simulink model "btp_VERSION2_draft1"  (R2020a)
settings: Solver=VariableStepAuto  StartTime=0.0  StopTime=1e5  RelTol=1e-3
PreLoadFcn:
  | building_length = 15; % m
  | building_width = 10; % m
  | building_height = 2.5; % m
  | 
  | wall_thickness = 0.2; % m
  | wall_density = 2000; % kg/m^3
  | wall_specific_heat = 840; % J/(kg*K)
  | wall_conductivity = 0.04; % W/(m*K)
  | wall_heat_transfer_coeff_internal = 25; % W/(m^2*K)
  | wall_heat_transfer_coeff_external = 35; % W/(m^2*K)
  | 
  | roof_thickness = 0.2; % m
  | roof_density = 2000; % kg/m^3
  | roof_specific_heat = 840; % J/(kg*K)
  | roof_conductivity = 0.035; % W/(m*K)
  | roof_heat_transfer_coeff_internal = 10; % W/(m^2*K)
  | roof_heat_transfer_coeff_external = 30; % W/(m^2*K)
  | 
  | floor_thickness = 0.1; % m
  | floor_conductivity = 0.15; % W/(m*K)
  | floor_heat_transfer_coeff_internal = 15; % W/(m^2*K)
  | 
  | door_area = 2*0.6; % m^2
  | 
  | duct_area = 0.1^2; % m^2
  | 
  | fan_setting_table = 0 : 4; % 1
  | fan_flow_rate_table = [0 0.08 0.12 0.16 0.2]; % kg/s
  | 
  | initial_temperature = 35; % degC
  | ground_temperature = 25; % degC
  | 
  | flow_reversal_Mach = 1e-5; % 1
InitFcn:
  | zone_volume = building_length * building_width * building_height / 4; % m^3
  | zone_flow_area = 0.7 * building_height * (building_length + building_width) / 4; % m^2
model workspace (MAT data in the model file):
  CO2_occupant = 0.01
  N_occupant = 1
  T_occupant = 30
  W_occupant = 70
  y_co2_env = 0.04
undefined symbols (not defined in the file): mdot_coolant, sigbuilder_block, T_coolant
libraries: fl_lib x57, nesl_utility x23, HVAC_lib x1
(part 1 of 2)
CloseFcn:
  | try,close(h1_ssc_building_ventilation),end
  | clear h1_ssc_building_ventilation
  | try,close(h2_ssc_building_ventilation),end
  | clear h2_ssc_building_ventilation
  | try,close(h3_ssc_building_ventilation),end
  | clear h3_ssc_building_ventilation
  | try,close(h4_ssc_building_ventilation),end
  | clear h4_ssc_building_ventilation
  | 
  | clear simlog_ssc_building_ventilation tout
  | 
  | clear building_length building_width building_height zone_volume zone_flow_area
  | clear wall_thickness wall_density wall_specific_heat wall_conductivity wall_heat_transfer_coeff_internal wall_heat_transfer_coeff_external
  | clear roof_thickness roof_density roof_specific_heat roof_conductivity roof_heat_transfer_coeff_internal roof_heat_transfer_coeff_external
  | clear floor_thickness floor_conductivity floor_heat_transfer_coeff_internal
  | clear door_area duct_area fan_setting_table fan_flow_rate_table initial_temperature ground_temperature flow_reversal_Mach
Description:
  | Building Ventilation
settings Model: Creator=MathWorks  LastModifiedBy=PRANAV REDDY
settings DataIOCC: ReturnWorkspaceOutputs=off
settings DebuggingCC: PregeneratedLibrarySubsystemCodeDiagnostic=none  ArithmeticOperatorsInVariantConditions=warning
settings SFSimCC: SimUseLocalCustomCode=off  CustomCodeUndefinedFunction=UseInterfaceOnly
settings RTWCC: RTWUseLocalCustomCode=off
settings CodeAppCC: StateflowObjectComments=on
settings SimscapeCC: SimscapeLogType=all  SimscapeLogSimulationStatistics=on  SimscapeLogName=simlog_ssc_building_ventilation  SimscapeLogDataHistory=10000

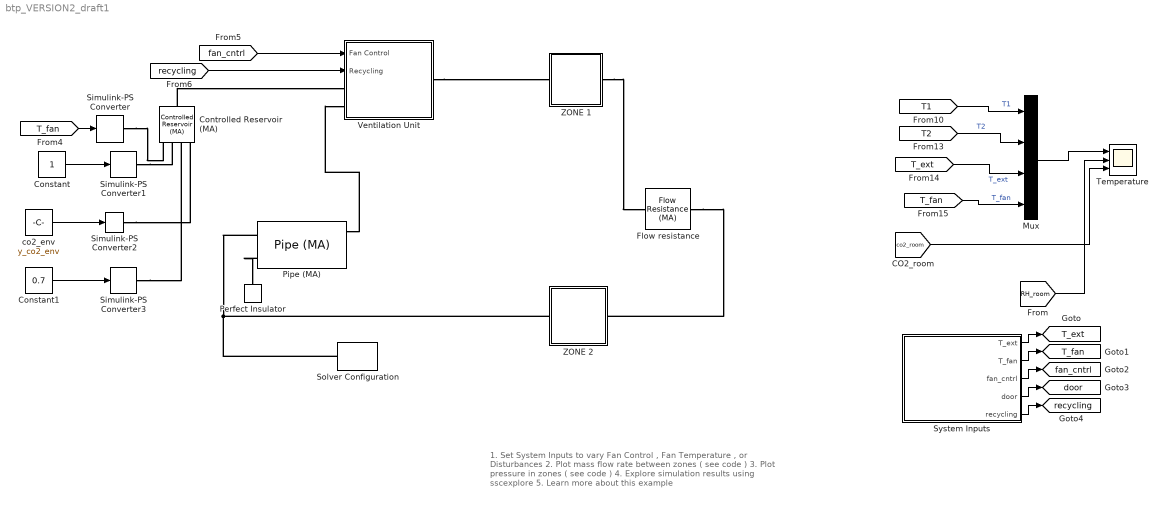
== system btp_VERSION2_draft1 ==
  note: 1. Set System Inputs to vary Fan Control , Fan Temperature , or Disturbances
      | 2. Plot mass flow rate between zones ( see code )
      | 3. Plot pressure in zones ( see code )
      | 4. Explore simulation results using sscexplore
      | 5. Learn more about this example
  Constant : Constant
  Constant1 : Constant  Value=0.7
  Controlled Reservoir (MA) : fl_lib/Moist Air/Elements/Controlled Reservoir (MA)  moisture_spec=foundation.enum.moisture_spec.relative_humidity  trace_gas_spec=foundation.enum.trace_gas_spec.mole_fraction  RH_ws=1  area_A=duct_area m^2  input_error_spec=foundation.enum.input_range_error.warn
      settings: SourceProductBaseCode=SS  InternalSimscapePortConfiguration="{\"Bottom\":[],\"Left\":[{\"id\":\"A\",\"label\":\"A\",\"type\":\"foundation.moist_air.moist_air\"}],\"Right\":[{\"id\":\"T\",\"label\":\"T\",\"type\":\"input\"},{\"id\":\"P\",\"label\":\"P\",\"type\":\"input\"},{\"id\":\"W\",\"label\":\"W\",\"type\":\"input\"},{\"id\":\"G\",\"label\":\"G\",\"type\":\"input\"}],\"Top\":[]}"
  Flow resistance : fl_lib/Moist Air/Elements/Flow Resistance (MA)  delta_p_nominal=20 Pa  mdot_nominal=0.04 kg/s  rho_nominal=1.2 kg/m^3  area=zone_flow_area m^2  laminar_fraction=1e-3
      settings: SourceProductBaseCode=SS
  Mux : Mux
  Perfect Insulator : fl_lib/Thermal/Thermal Elements/Perfect Insulator  T_specify=off  T_priority=None  T=0 K  T_nominal_specify=off  T_nominal_unit=K  T_nominal_value=1
  Pipe (MA) : fl_lib/Moist Air/Elements/Pipe (MA)  length=building_length + building_width m  area=duct_area m^2  Dh=sqrt(duct_area) m  length_add=0 m  roughness=15e-6 m  Re_lam=2000  Re_tur=4000  shape_factor=56.92  Nu_lam=2.98  RH_ws=1  time_constant=1e-3 s  moisture_trace_gas_source=foundation.enum.moisture_trace_gas_source.none  moisture_source_spec=foundation.enum.moisture_source_spec.vapor  moisture_mass_flow=0 kg/s  moisture_temperature_spec=foundation.enum.temperature_spec.atmospheric  moisture_temperature=293.15 K  trace_gas_mass_flow=0 kg/s  trace_gas_temperature_spec=foundation.enum.temperature_spec.atmospheric  trace_gas_temperature=293.15 K  p_I_specify=off  p_I_priority=High  p_I=0.101325 MPa  p_I_nominal_specify=off  p_I_nominal_unit=MPa  p_I_nominal_value=1  T_I_specify=off  T_I_priority=High  T_I=293.15 K  T_I_nominal_specify=off  T_I_nominal_unit=K  T_I_nominal_value=1  RH_I_specify=off  RH_I_priority=High  RH_I=0  RH_I_nominal_specify=off  RH_I_nominal_unit=1  RH_I_nominal_value=1  x_w_I_specify=off  x_w_I_priority=None  x_w_I=0  x_w_I_nominal_specify=off  x_w_I_nominal_unit=1  x_w_I_nominal_value=1  y_w_I_specify=off  y_w_I_priority=None  y_w_I=0  y_w_I_nominal_specify=off  y_w_I_nominal_unit=1  y_w_I_nominal_value=1  HR_I_specify=off  HR_I_priority=None  HR_I=0  HR_I_nominal_specify=off  HR_I_nominal_unit=1  HR_I_nominal_value=1  x_g_I_specify=off  x_g_I_priority=High  x_g_I=0  x_g_I_nominal_specify=off  x_g_I_nominal_unit=1  x_g_I_nominal_value=1  y_g_I_specify=off  y_g_I_priority=None  y_g_I=0  y_g_I_nominal_specify=off  y_g_I_nominal_unit=1  y_g_I_nominal_value=1
      settings: SourceProductBaseCode=SS
  Simulink-PS Converter : nesl_utility/Simulink-PS Converter  PhysicalDomain=network_engine_domain  SubClassName=ps_input  LeftPortType=input  RightPortType=output  PseudoPeriodic=off  Frequencies=[]  NoiseDistribution=none  NoiseParameters=[]  Unit=degC  AffineConversion=on  FilteringAndDerivatives=provide  SimscapeFilterOrder=1  InputFilterTimeConstant=0.001  UdotUserProvided=0
  Simulink-PS Converter1 : nesl_utility/Simulink-PS Converter  PhysicalDomain=network_engine_domain  SubClassName=ps_input  LeftPortType=input  RightPortType=output  PseudoPeriodic=off  Frequencies=[]  NoiseDistribution=none  NoiseParameters=[]  Unit=atm  AffineConversion=off  FilteringAndDerivatives=provide  SimscapeFilterOrder=1  InputFilterTimeConstant=0.001  UdotUserProvided=0
  Simulink-PS Converter2 : nesl_utility/Simulink-PS Converter  PhysicalDomain=network_engine_domain  SubClassName=ps_input  LeftPortType=input  RightPortType=output  PseudoPeriodic=off  Frequencies=[]  NoiseDistribution=none  NoiseParameters=[]  Unit=1  AffineConversion=off  FilteringAndDerivatives=provide  SimscapeFilterOrder=1  InputFilterTimeConstant=0.001  UdotUserProvided=0
  Simulink-PS Converter3 : nesl_utility/Simulink-PS Converter  PhysicalDomain=network_engine_domain  SubClassName=ps_input  LeftPortType=input  RightPortType=output  PseudoPeriodic=off  Frequencies=[]  NoiseDistribution=none  NoiseParameters=[]  Unit=1  AffineConversion=off  FilteringAndDerivatives=provide  SimscapeFilterOrder=1  InputFilterTimeConstant=0.001  UdotUserProvided=0
  Solver Configuration : nesl_utility/Solver Configuration  PhysicalDomain=network_engine_domain  SubClassName=solver  LeftPortType=input  RightPortType=generic  Tones=[]  Harmonics=[]  SimulateNoise=off  Profile=off  UseLocalSampling=off  EnableSwitchedLinearOptims=on  FrequencyDomain=off  UseCCode=off  RelTol=0.001  AbsTol=1e-06  MinStep=1e-09  ToWorkspace=off  RevertToSquareIcSolve=off  NumHomotopyIterations=100  PhasorMode=off  PhasorModeNumHarmonics=1  DoDC=off  ResidualTolerance=1e-9  UseLocalSolver=off  LocalSolverChoice=NE_BACKWARD_EULER_ADVANCER  LocalSolverSampleTime=0.05  DoFixedCost=off  MaxNonlinIter=3  MaxModeIter=2  LinearAlgebra=auto  EquationFormulation=NE_TIME_EF  DelaysMemoryBudget=1024  AutomaticFiltering=on  FilteringTimeConstant=0.001  PartitionStorageMethod=AS_NEEDED  PartitionMemoryBudget=1024  PartitionMethod=FAST
  System Inputs : Subsystem  Tag=STV Subsys  LoadFcn=sigbuilder_block('load');  StartFcn=sigbuilder_block('start');  StopFcn=sigbuilder_block('stop');  ClipboardFcn=sigbuilder_block('clipboard');  mask(Sigbuilder block){tuvar=[0:10]}
      mask help: Simulink:masks:SigbuilderBlock_MD
      mask init:
      | if ~strcmp(get_param(bdroot(gcbh),'SimulationStatus'),'stopped') tuvar = sigbuilder_block('maskInit'); end
      settings: CopyFcn=sigbuilder_block('copy');  DeleteFcn=sigbuilder_block('delete');  ModelCloseFcn=sigbuilder_block('modelClose');  PreSaveFcn=sigbuilder_block('preSave');  PauseFcn=sigbuilder_block('pause');  ContinueFcn=sigbuilder_block('continue');  NameChangeFcn=sigbuilder_block('namechange');  OpenFcn=sigbuilder_block('open',[96 153 550.5 359.25 ]);  CloseFcn=sigbuilder_block('close');
      mask Display: plot(0, 0, 100, 100,[2, 2, 32, 32, 2], [68, 8, 8, 68, 68],[32, 2], [38, 38], [32, 19, 2],[53, 60, 44], [32, 17, 17, 2],[16, 16, 31, 31]);txt = getActiveGroup(gcbh);text(2, 100, txt,'verticalAlignment', 'top');
  Temperature : Scope  NumInputPorts=3
  Ventilation Unit : Subsystem  Tag=PublishSubsystem
  ZONE 1 : Subsystem
  ZONE 2 : Subsystem
  co2_env : Constant  Value=y_co2_env
  tag scope: T_ext=global, T_fan=global, door=global, fan_cntrl=global, recycling=global
  wires:
  Constant/1 -> Simulink-PS Converter1/1
  [T_fan] -> Simulink-PS Converter/1
  [fan_cntrl] -> Ventilation Unit/1(Fan Control)
  [recycling] -> Ventilation Unit/2(Recycling)
  System Inputs/1(T_ext) -> [T_ext]
  System Inputs/2(T_fan) -> [T_fan]
  System Inputs/3(fan_cntrl) -> [fan_cntrl]
  System Inputs/4(door) -> [door]
  System Inputs/5(recycling) -> [recycling]
  [T1] -> Mux/1  "T1"
  [T2] -> Mux/2  "T2"
  [T_ext] -> Mux/3  "T_ext"
  [T_fan] -> Mux/4  "T_fan"
  Mux/1 -> Temperature/1
  co2_env/1 -> Simulink-PS Converter2/1
  [co2_room] -> Temperature/3
  Constant1/1 -> Simulink-PS Converter3/1
  [RH_room] -> Temperature/2
  connections:
  Simulink-PS Converter/RConn1 -- Controlled Reservoir (MA)/RConn1
  Simulink-PS Converter1/RConn1 -- Controlled Reservoir (MA)/RConn2
  Controlled Reservoir (MA)/LConn1 -- Ventilation Unit/LConn1
  Pipe (MA)/RConn1 -- Ventilation Unit/LConn2
  Pipe (MA)/LConn2 -- Perfect Insulator/LConn1
  Solver Configuration/RConn1 -- Pipe (MA)/LConn1 -- ZONE 2/LConn1
  Flow resistance/RConn1 -- ZONE 2/RConn1
  ZONE 1/RConn1 -- Flow resistance/LConn1
  Ventilation Unit/RConn1 -- ZONE 1/LConn1
  Simulink-PS Converter2/RConn1 -- Controlled Reservoir (MA)/RConn4
  Simulink-PS Converter3/RConn1 -- Controlled Reservoir (MA)/RConn3

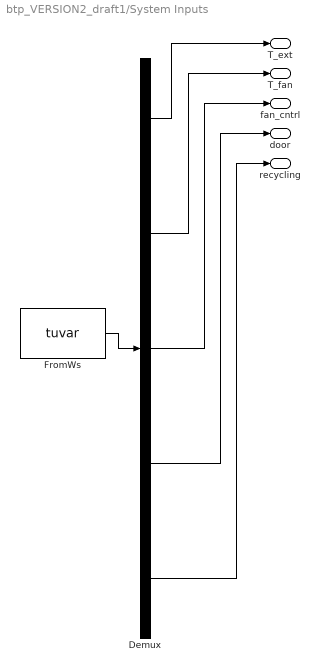
== system btp_VERSION2_draft1/System Inputs ==
  Demux : Demux  Tag=STV Demux  Outputs=5
      settings: DisplayOption=none
  FromWs : FromWorkspace  Tag=STV FromWs  VariableName=tuvar
      SigBuilderData=|
      | common.afterFinalStr = 'Extrapolate'
      | common.sampleTime = 0
      | dataSet(1).timeRange = [0 100000]
      | dataSet(1).name = 'Fan Control'
      | dataSet(2).timeRange = [0 100000]
      | dataSet(2).name = 'Fan Temperature'
      | dataSet(3).timeRange = [0 100000]
      | dataSet(3).name = 'Disturbances'
      | sbobj.Groups(1).Name = 'Fan Control'
      | sbobj.Groups(1).Signals(1).Name = 'T_ext'
      | sbobj.Groups(1).Signals(1).XData = [0 100000]
      | sbobj.Groups(1).Signals(1).YData = [35 35]
      | sbobj.Groups(1).Signals(2).Name = 'T_fan'
      | sbobj.Groups(1).Signals(2).XData = [0 100000]
      | sbobj.Groups(1).Signals(2).YData = [20 20]
      | sbobj.Groups(1).Signals(3).Name = 'fan_cntrl'
      | sbobj.Groups(1).Signals(3).XData = [0 20000 20000 40000 40000 60000 60000 80000 80000 100000]
      | sbobj.Groups(1).Signals(3).YData = [1 1 2 2 1 1 0 0 1 1]
      | sbobj.Groups(1).Signals(4).Name = 'door'
      | sbobj.Groups(1).Signals(4).XData = [0 100000]
      | sbobj.Groups(1).Signals(4).YData = [0 0]
      | sbobj.Groups(1).Signals(5).Name = 'recycling'
      | sbobj.Groups(1).Signals(5).XData = [0 100000]
      | sbobj.Groups(1).Signals(5).YData = [0 0]
      | sbobj.Groups(1).TimeRange = [0 100000]
      | sbobj.Groups(2).Name = 'Fan Temperature'
      | sbobj.Groups(2).Signals(1).Name = 'T_ext'
      | sbobj.Groups(2).Signals(1).XData = [0 100000]
      | sbobj.Groups(2).Signals(1).YData = [35 35]
      | sbobj.Groups(2).Signals(2).Name = 'T_fan'
      | sbobj.Groups(2).Signals(2).XData = [0 20000 40000 60000 80000 100000]
      | sbobj.Groups(2).Signals(2).YData = [20 20 20 20 20 20]
      | sbobj.Groups(2).Signals(3).Name = 'fan_cntrl'
      | sbobj.Groups(2).Signals(3).XData = [0 100000]
      | sbobj.Groups(2).Signals(3).YData = [1 1]
      | sbobj.Groups(2).Signals(4).Name = 'door'
      | sbobj.Groups(2).Signals(4).XData = [0 24200 34000 43600 100000]
      | sbobj.Groups(2).Signals(4).YData = [0 0 1.1 0 0]
      | sbobj.Groups(2).Signals(5).Name = 'recycling'
      | sbobj.Groups(2).Signals(5).XData = [0 20400 20400 78000 78000 100000]
      | sbobj.Groups(2).Signals(5).YData = [0 0 1 1 0 0]
      | sbobj.Groups(2).TimeRange = [0 100000]
      | sbobj.Groups(3).Name = 'Disturbances'
      | sbobj.Groups(3).Signals(1).Name = 'T_ext'
      | sbobj.Groups(3).Signals(1).XData = [0 100000]
      | sbobj.Groups(3).Signals(1).YData = [33.8 33.8]
      | sbobj.Groups(3).Signals(2).Name = 'T_fan'
      | sbobj.Groups(3).Signals(2).XData = [0 100000]
      | sbobj.Groups(3).Signals(2).YData = [21 21]
      | sbobj.Groups(3).Signals(3).Name = 'fan_cntrl'
      | sbobj.Groups(3).Signals(3).XData = [0 100000]
      | sbobj.Groups(3).Signals(3).YData = [1 1]
      | sbobj.Groups(3).Signals(4).Name = 'door'
      | sbobj.Groups(3).Signals(4).XData = [0 20000 30000 40000 100000]
      | sbobj.Groups(3).Signals(4).YData = [0 0 1 0 0]
      | sbobj.Groups(3).Signals(5).Name = 'recycling'
      | sbobj.Groups(3).Signals(5).XData = [0 65800 65800 95400 95400 100000]
      | sbobj.Groups(3).Signals(5).YData = [0 0 1 1 0 0]
      | sbobj.Groups(3).TimeRange = [0 100000]
  T_ext : Outport  Tag=STV Outport  VectorParamsAs1DForOutWhenUnconnected=off
  T_fan : Outport  Tag=STV Outport  Port=2  VectorParamsAs1DForOutWhenUnconnected=off
  fan_cntrl : Outport  Tag=STV Outport  Port=3  VectorParamsAs1DForOutWhenUnconnected=off
  door : Outport  Tag=STV Outport  Port=4  VectorParamsAs1DForOutWhenUnconnected=off
  recycling : Outport  Tag=STV Outport  Port=5  VectorParamsAs1DForOutWhenUnconnected=off
  wires:
  FromWs/1 -> Demux/1
  Demux/1 -> T_ext/1
  Demux/2 -> T_fan/1
  Demux/3 -> fan_cntrl/1
  Demux/4 -> door/1
  Demux/5 -> recycling/1

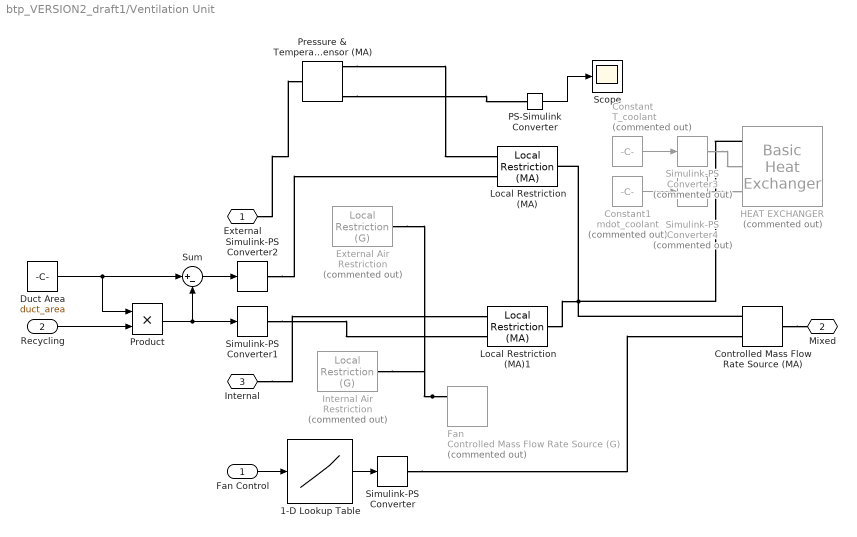
== system btp_VERSION2_draft1/Ventilation Unit ==
  Fan Control : Inport
  Recycling : Inport  Port=2
  1-D Lookup Table : Lookup_n-D  NumberOfTableDimensions=1  BreakpointsForDimension1=fan_setting_table  Table=fan_flow_rate_table  ExtrapMethod=Clip  InternalRulePriority=Speed  RndMeth=Simplest  InputSameDT=on
  Constant : Constant  Commented=on  Value=T_coolant
  Constant1 : Constant  Commented=on  Value=mdot_coolant
  Controlled Mass Flow Rate Source (MA) : fl_lib/Moist Air/Sources/Controlled Mass Flow Rate Source (MA)  power_spec=foundation.enum.power_spec.isentropic  area_A=duct_area m^2  area_B=duct_area m^2
      settings: SourceProductBaseCode=SS  InternalSimscapePortConfiguration="{\"Bottom\":[],\"Left\":[{\"id\":\"A\",\"label\":\"A\",\"type\":\"foundation.moist_air.moist_air\"},{\"id\":\"M\",\"label\":\"M\",\"type\":\"input\"}],\"Right\":[{\"id\":\"B\",\"label\":\"B\",\"type\":\"foundation.moist_air.moist_air\"}],\"Top\":[]}"
  Duct Area : Constant  Value=duct_area
  External Air Restriction : fl_lib/Gas/Elements/Local Restriction (G)  Commented=on  restriction_type=foundation.enum.restriction_type.variable  restriction_area=1e-3 m^2  min_area=1e-10 m^2  max_area=0.99 * duct_area m^2  area=duct_area m^2  Cd=0.8  B_lam=0.999
      settings: SourceProductBaseCode=SS  InternalSimscapePortConfiguration="{\"Bottom\":[],\"Left\":[{\"id\":\"A\",\"label\":\"A\",\"type\":\"foundation.gas.gas\"},{\"id\":\"area_in\",\"label\":\"AR\",\"type\":\"input\"}],\"Right\":[{\"id\":\"B\",\"label\":\"B\",\"type\":\"foundation.gas.gas\"}],\"Top\":[]}"
  Fan : fl_lib/Gas/Sources/Controlled Mass Flow Rate Source (G)  Commented=on  power_spec=1  area_A=duct_area m^2  area_B=duct_area m^2
      settings: SourceProductName=Foundation Library  InternalSimscapePortConfiguration="{\"Bottom\":[],\"Left\":[{\"id\":\"A\",\"label\":\"A\",\"type\":\"foundation.gas.gas\"},{\"id\":\"M\",\"label\":\"M\",\"type\":\"input\"}],\"Right\":[{\"id\":\"B\",\"label\":\"B\",\"type\":\"foundation.gas.gas\"}],\"Top\":[]}"
  HEAT EXCHANGER : HVAC_lib/Basic Heat Exchanger  Commented=on  Q_des=4.8 kW  T1_des=30 degC  mdot1_des=3 kg/s  cp1_des=1.8 kJ/kg/K  Dp1_des=0.2 kPa  T2_des=T_coolant degC  mdot2_des=mdot_coolant kg/s  cp2_des=10 kJ/kg/K  volume=1e-1 m^3  port_area=duct_area m^2  RH_ws=1  time_constant=1e-3 s  p_I_specify=on  p_I_priority=High  p_I=p_env MPa  p_I_nominal_specify=off  p_I_nominal_unit=MPa  p_I_nominal_value=1  T_I_specify=on  T_I_priority=High  T_I=T_init degC  T_I_nominal_specify=off  T_I_nominal_unit=K  T_I_nominal_value=1  RH_I_specify=on  RH_I_priority=High  RH_I=RH_init  RH_I_nominal_specify=off  RH_I_nominal_unit=1  RH_I_nominal_value=1  x_w_I_specify=off  x_w_I_priority=None  x_w_I=0  x_w_I_nominal_specify=off  x_w_I_nominal_unit=1  x_w_I_nominal_value=1  y_w_I_specify=off  y_w_I_priority=None  y_w_I=0  y_w_I_nominal_specify=off  y_w_I_nominal_unit=1  y_w_I_nominal_value=1  HR_I_specify=off  HR_I_priority=None  HR_I=0  HR_I_nominal_specify=off  HR_I_nominal_unit=1  HR_I_nominal_value=1  x_g_I_specify=on  x_g_I_priority=None  x_g_I=0  x_g_I_nominal_specify=off  x_g_I_nominal_unit=1  x_g_I_nominal_value=1  y_g_I_specify=on  y_g_I_priority=High  y_g_I=y_CO2_env  y_g_I_nominal_specify=off  y_g_I_nominal_unit=1  y_g_I_nominal_value=1
      settings: SourceProductBaseCode=SS  InternalSimscapePortConfiguration="{\"Bottom\":[],\"Left\":[{\"id\":\"A\",\"label\":\"A\",\"type\":\"foundation.moist_air.moist_air\"},{\"id\":\"T2\",\"label\":\"T2\",\"type\":\"input\"},{\"id\":\"M2\",\"label\":\"M2\",\"type\":\"input\"}],\"Right\":[{\"id\":\"B\",\"label\":\"B\",\"type\":\"foundation.moist_air.moist_air\"},{\"id\":\"W\",\"label\":\"W\",\"type\":\"output\"},{\"id\":\"F\",\"label\":\"F\",\"type\":\"output\"}],\"Top\":[]}"
  Internal Air Restriction : fl_lib/Gas/Elements/Local Restriction (G)  Commented=on  restriction_type=foundation.enum.restriction_type.variable  restriction_area=1e-3 m^2  min_area=1e-10 m^2  max_area=0.99 * duct_area m^2  area=duct_area m^2  Cd=0.8  B_lam=0.999
      settings: SourceProductBaseCode=SS  InternalSimscapePortConfiguration="{\"Bottom\":[],\"Left\":[{\"id\":\"A\",\"label\":\"A\",\"type\":\"foundation.gas.gas\"},{\"id\":\"area_in\",\"label\":\"AR\",\"type\":\"input\"}],\"Right\":[{\"id\":\"B\",\"label\":\"B\",\"type\":\"foundation.gas.gas\"}],\"Top\":[]}"
  Local Restriction (MA) : fl_lib/Moist Air/Elements/Local Restriction (MA)  restriction_type=foundation.enum.restriction_type.variable  restriction_area=0.001 m^2  min_area=1e-10 m^2  max_area=0.99*duct_area m^2  area=duct_area m^2  Cd=0.8  B_lam=0.999
      settings: SourceProductBaseCode=SS
  Local Restriction (MA)1 : fl_lib/Moist Air/Elements/Local Restriction (MA)  restriction_type=foundation.enum.restriction_type.variable  restriction_area=0.001 m^2  min_area=1e-10 m^2  max_area=0.99 * duct_area m^2  area=duct_area m^2  Cd=0.8  B_lam=0.999
      settings: SourceProductBaseCode=SS
  PS-Simulink Converter : nesl_utility/PS-Simulink Converter  PhysicalDomain=network_engine_domain  SubClassName=ps_output  LeftPortType=input  RightPortType=output  PseudoPeriodic=off  Frequencies=[]  Unit=inherit  AffineConversion=off
  Pressure & Temperature Sensor (MA) : fl_lib/Moist Air/Sensors/Pressure & Temperature Sensor (MA)
      settings: SourceProductBaseCode=SS  InternalSimscapePortConfiguration="{\"Bottom\":[],\"Left\":[{\"id\":\"A\",\"label\":\"A\",\"type\":\"foundation.moist_air.moist_air\"}],\"Right\":[{\"id\":\"B\",\"label\":\"B\",\"type\":\"foundation.moist_air.moist_air\"},{\"id\":\"P\",\"label\":\"P\",\"type\":\"output\"},{\"id\":\"T\",\"label\":\"T\",\"type\":\"output\"}],\"Top\":[]}"
  Product : Product
  Scope : Scope
  Simulink-PS Converter : nesl_utility/Simulink-PS Converter  PhysicalDomain=network_engine_domain  SubClassName=ps_input  LeftPortType=input  RightPortType=output  PseudoPeriodic=off  Frequencies=[]  NoiseDistribution=none  NoiseParameters=[]  Unit=kg/s  AffineConversion=off  FilteringAndDerivatives=provide  SimscapeFilterOrder=1  InputFilterTimeConstant=0.001  UdotUserProvided=0
  Simulink-PS Converter1 : nesl_utility/Simulink-PS Converter  PhysicalDomain=network_engine_domain  SubClassName=ps_input  LeftPortType=input  RightPortType=output  PseudoPeriodic=off  Frequencies=[]  NoiseDistribution=none  NoiseParameters=[]  Unit=m^2  AffineConversion=off  FilteringAndDerivatives=provide  SimscapeFilterOrder=1  InputFilterTimeConstant=0.001  UdotUserProvided=0
  Simulink-PS Converter2 : nesl_utility/Simulink-PS Converter  PhysicalDomain=network_engine_domain  SubClassName=ps_input  LeftPortType=input  RightPortType=output  PseudoPeriodic=off  Frequencies=[]  NoiseDistribution=none  NoiseParameters=[]  Unit=m^2  AffineConversion=off  FilteringAndDerivatives=provide  SimscapeFilterOrder=1  InputFilterTimeConstant=0.001  UdotUserProvided=0
  Simulink-PS Converter3 : nesl_utility/Simulink-PS Converter  Commented=on  PhysicalDomain=network_engine_domain  SubClassName=ps_input  LeftPortType=input  RightPortType=output  PseudoPeriodic=off  Frequencies=[]  NoiseDistribution=none  NoiseParameters=[]  Unit=degC  AffineConversion=off  FilteringAndDerivatives=provide  SimscapeFilterOrder=1  InputFilterTimeConstant=0.001  UdotUserProvided=0
  Simulink-PS Converter4 : nesl_utility/Simulink-PS Converter  Commented=on  PhysicalDomain=network_engine_domain  SubClassName=ps_input  LeftPortType=input  RightPortType=output  PseudoPeriodic=off  Frequencies=[]  NoiseDistribution=none  NoiseParameters=[]  Unit=kg/s  AffineConversion=on  FilteringAndDerivatives=provide  SimscapeFilterOrder=1  InputFilterTimeConstant=0.001  UdotUserProvided=0
  Sum : Sum  Inputs=|+-
  External : PMIOPort  Side=Left
  Mixed : PMIOPort  Port=2  Side=Right
  Internal : PMIOPort  Port=3  Side=Left
  wires:
  Fan Control/1 -> 1-D Lookup Table/1
  1-D Lookup Table/1 -> Simulink-PS Converter/1
  Recycling/1 -> Product/2
  Product/1 -> Sum/2, Simulink-PS Converter1/1
  Sum/1 -> Simulink-PS Converter2/1
  Duct Area/1 -> Sum/1, Product/1
  Constant1/1 -> Simulink-PS Converter4/1
  Constant/1 -> Simulink-PS Converter3/1
  PS-Simulink Converter/1 -> Scope/1
  connections:
  Simulink-PS Converter/RConn1 -- Controlled Mass Flow Rate Source (MA)/LConn2
  Fan/LConn1 -- Internal Air Restriction/RConn1 -- External Air Restriction/RConn1
  External/RConn1 -- Pressure & Temperature Sensor (MA)/LConn1
  Simulink-PS Converter2/RConn1 -- Local Restriction (MA)/LConn2
  Controlled Mass Flow Rate Source (MA)/RConn1 -- Mixed/RConn1
  Simulink-PS Converter1/RConn1 -- Local Restriction (MA)1/LConn2
  Internal/RConn1 -- Local Restriction (MA)1/LConn1
  Local Restriction (MA)1/RConn1 -- Controlled Mass Flow Rate Source (MA)/LConn1 -- HEAT EXCHANGER/LConn1 -- Local Restriction (MA)/RConn1
  Simulink-PS Converter3/RConn1 -- HEAT EXCHANGER/LConn2
  Simulink-PS Converter4/RConn1 -- HEAT EXCHANGER/LConn3
  Pressure & Temperature Sensor (MA)/RConn1 -- Local Restriction (MA)/LConn1
  Pressure & Temperature Sensor (MA)/RConn3 -- PS-Simulink Converter/LConn1

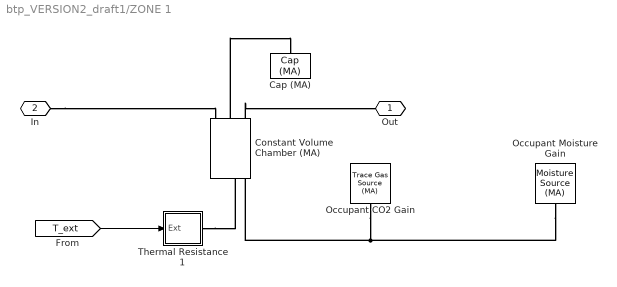
== system btp_VERSION2_draft1/ZONE 1 ==
  Cap (MA) : fl_lib/Moist Air/Elements/Cap (MA)  p_specify=off  p_priority=None  p=0.101325 MPa  p_nominal_specify=off  p_nominal_unit=MPa  p_nominal_value=1  T_specify=off  T_priority=None  T=293.15 K  T_nominal_specify=off  T_nominal_unit=K  T_nominal_value=1  x_w_specify=off  x_w_priority=None  x_w=0  x_w_nominal_specify=off  x_w_nominal_unit=1  x_w_nominal_value=1  x_g_specify=off  x_g_priority=None  x_g=0  x_g_nominal_specify=off  x_g_nominal_unit=1  x_g_nominal_value=1
      settings: SourceProductBaseCode=SS  InternalSimscapePortConfiguration="{\"Bottom\":[],\"Left\":[{\"id\":\"A\",\"label\":\"\",\"type\":\"foundation.moist_air.moist_air\"}],\"Right\":[],\"Top\":[]}"
  Constant Volume Chamber (MA) : fl_lib/Moist Air/Elements/Constant Volume Chamber (MA)  volume=zone_volume m^3  num_ports=foundation.enum.num_ports.three  area_A=duct_area m^2  area_B=zone_flow_area m^2  area_C=zone_flow_area m^2  area_D=0.01 m^2  RH_ws=1  time_constant=1e-3 s  moisture_trace_gas_source=foundation.enum.moisture_trace_gas_source.controlled  moisture_source_spec=foundation.enum.moisture_source_spec.vapor  moisture_mass_flow=0 kg/s  moisture_temperature_spec=foundation.enum.temperature_spec.atmospheric  moisture_temperature=293.15 K  trace_gas_mass_flow=0 kg/s  trace_gas_temperature_spec=foundation.enum.temperature_spec.atmospheric  trace_gas_temperature=293.15 K  p_I_specify=off  p_I_priority=High  p_I=0.101325 MPa  p_I_nominal_specify=off  p_I_nominal_unit=MPa  p_I_nominal_value=1  T_I_specify=off  T_I_priority=High  T_I=300 K  T_I_nominal_specify=off  T_I_nominal_unit=K  T_I_nominal_value=1  RH_I_specify=off  RH_I_priority=High  RH_I=0  RH_I_nominal_specify=off  RH_I_nominal_unit=1  RH_I_nominal_value=1  x_w_I_specify=off  x_w_I_priority=None  x_w_I=0  x_w_I_nominal_specify=off  x_w_I_nominal_unit=1  x_w_I_nominal_value=1  y_w_I_specify=off  y_w_I_priority=None  y_w_I=0  y_w_I_nominal_specify=off  y_w_I_nominal_unit=1  y_w_I_nominal_value=1  HR_I_specify=off  HR_I_priority=None  HR_I=0  HR_I_nominal_specify=off  HR_I_nominal_unit=1  HR_I_nominal_value=1  x_g_I_specify=off  x_g_I_priority=High  x_g_I=0  x_g_I_nominal_specify=off  x_g_I_nominal_unit=1  x_g_I_nominal_value=1  y_g_I_specify=off  y_g_I_priority=None  y_g_I=300  y_g_I_nominal_specify=off  y_g_I_nominal_unit=1  y_g_I_nominal_value=1
      settings: SourceProductBaseCode=SS  InternalSimscapePortConfiguration="{\"Bottom\":[],\"Left\":[{\"id\":\"A\",\"label\":\"A\",\"type\":\"foundation.moist_air.moist_air\"},{\"id\":\"B\",\"label\":\"B\",\"type\":\"foundation.moist_air.moist_air\"},{\"id\":\"C\",\"label\":\"C\",\"type\":\"foundation.moist_air.moist_air\"}],\"Right\":[{\"id\":\"W\",\"label\":\"W\",\"type\":\"output\"},{\"id\":\"F\",\"label\":\"F\",\"type\":\"output\"},{\"id\":\"H\",\"label\":\"H\",\"type\":\"foundation.thermal.thermal\"},{\"id\":\"S\",\"label\":\"S\",\"type\":\"foundation.moist_air.moist_air_source\"}],\"Top\":[]}"
  Occupant CO2 Gain : fl_lib/Moist Air/Sources/Moisture & Trace Gas Sources/Trace Gas Source (MA)  trace_gas_mass_flow=CO2_occupant * N_occupant g/s  temperature_spec=2  trace_gas_temperature=T_occupant degC
      settings: SourceProductBaseCode=SS  InternalSimscapePortConfiguration="{\"Bottom\":[],\"Left\":[{\"id\":\"S\",\"label\":\"S\",\"type\":\"foundation.moist_air.moist_air_source\"}],\"Right\":[],\"Top\":[]}"
  Occupant Moisture Gain : fl_lib/Moist Air/Sources/Moisture & Trace Gas Sources/Moisture Source (MA)  moisture_source_spec=foundation.enum.moisture_source_spec.vapor  moisture_mass_flow=W_occupant * N_occupant g/s  temperature_spec=2  moisture_temperature=T_occupant degC
      settings: SourceProductBaseCode=SS  InternalSimscapePortConfiguration="{\"Bottom\":[],\"Left\":[{\"id\":\"S\",\"label\":\"S\",\"type\":\"foundation.moist_air.moist_air_source\"}],\"Right\":[],\"Top\":[]}"
  Thermal Resistance 1 : Subsystem  Tag=PublishSubsystem  mask(Zone Thermal Resistance){zone_length=building_length / 2, zone_width=building_width / 2, zone_height=building_height / 2, wall_thickness=wall_thickness, wall_density=wall_density, wall_specific_heat=wall_specific_heat, wall_conductivity=wall_conductivity, wall_heat_transfer_coeff_internal=wall_heat_transfer_coeff_internal, wall_heat_transfer_coeff_external=wall_heat_transfer_coeff_external, wall_initial_temperature=initial_temperature, roof_thickness=roof_thickness, roof_density=roof_density, roof_specific_heat=roof_specific_heat, roof_conductivity=roof_conductivity, roof_heat_transfer_coeff_internal=roof_heat_transfer_coeff_internal, roof_heat_transfer_coeff_external=roof_heat_transfer_coeff_external, roof_initial_temperature=initial_temperature, floor_thickness=floor_thickness, floor_conductivity=floor_conductivity, floor_heat_transfer_coeff_internal=floor_heat_transfer_coeff_internal, ground_temperature=ground_temperature}
      mask prompts: zone_length "Zone length (m)"; zone_width "Zone width (m)"; zone_height "Zone height (m)"; wall_thickness "Thickness (m)"; wall_density "Density (kg/m^3)"; wall_specific_heat "Specific heat (J/(kg*K))"; wall_conductivity "Thermal conductivity (W/(m*K))"; wall_heat_transfer_coeff_internal "Internal heat transfer coefficient (W/(m^2*K))"; wall_heat_transfer_coeff_external "External heat transfer coefficient (W/(m^2*K))"; wall_initial_temperature "Initial temperature (degC)"; roof_thickness "Thickness (m)"; roof_density "Density (kg/m^3)"; roof_specific_heat "Specific heat (J/(kg*K))"; roof_conductivity "Thermal conductivity (W/(m*K))"; roof_heat_transfer_coeff_internal "Internal heat transfer coefficient (W/(m^2*K))"; roof_heat_transfer_coeff_external "External heat transfer coefficient (W/(m^2*K))"; roof_initial_temperature "Initial temperature (degC)"; floor_thickness "Thickness (m)"; floor_conductivity "Thermal conductivity (W/(m*K))"; floor_heat_transfer_coeff_internal "Internal heat transfer coefficient (W/(m^2*K))"; ground_temperature "Ground temperature (degC)"
      mask help: This subsystem models the thermal resistances of the wall and of the roof between the zone and the external environment. It also models the thermal resistance of the floor between the zone and the ground.
      mask init:
      | wall_area = zone_height * (zone_length + zone_width);
      | roof_area = zone_length * zone_width;
      | floor_area = zone_length * zone_width;
      mask DialogControl TabGeometry Prompt: Geometry
      mask DialogControl TabWall Prompt: Wall
      mask DialogControl TabRoof Prompt: Roof
      mask DialogControl TabFloor Prompt: Floor
  Out : PMIOPort  Side=Right
  In : PMIOPort  Port=2  Side=Left
  wires:
  [T_ext] -> Thermal Resistance 1/1(Ext)
  connections:
  Occupant Moisture Gain/LConn1 -- Occupant CO2 Gain/LConn1 -- Constant Volume Chamber (MA)/RConn4
  Constant Volume Chamber (MA)/LConn2 -- Cap (MA)/LConn1
  In/RConn1 -- Constant Volume Chamber (MA)/LConn1
  Constant Volume Chamber (MA)/LConn3 -- Out/RConn1
  Thermal Resistance 1/RConn1 -- Constant Volume Chamber (MA)/RConn3

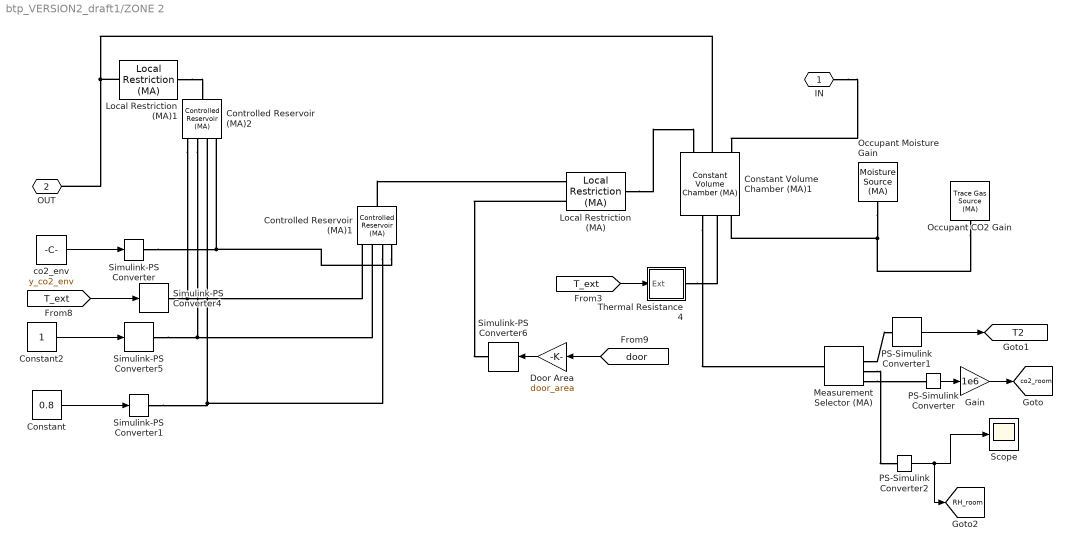
== system btp_VERSION2_draft1/ZONE 2 ==
  Constant : Constant  Value=0.8
  Constant Volume Chamber (MA)1 : fl_lib/Moist Air/Elements/Constant Volume Chamber (MA)  volume=zone_volume m^3  num_ports=foundation.enum.num_ports.three  area_A=duct_area m^2  area_B=zone_flow_area m^2  area_C=zone_flow_area m^2  area_D=0.01 m^2  RH_ws=1  time_constant=1e-3 s  moisture_trace_gas_source=foundation.enum.moisture_trace_gas_source.controlled  moisture_source_spec=foundation.enum.moisture_source_spec.vapor  moisture_mass_flow=0 kg/s  moisture_temperature_spec=foundation.enum.temperature_spec.atmospheric  moisture_temperature=293.15 K  trace_gas_mass_flow=0 kg/s  trace_gas_temperature_spec=foundation.enum.temperature_spec.atmospheric  trace_gas_temperature=293.15 K  p_I_specify=off  p_I_priority=High  p_I=0.101325 MPa  p_I_nominal_specify=off  p_I_nominal_unit=MPa  p_I_nominal_value=1  T_I_specify=off  T_I_priority=High  T_I=300 K  T_I_nominal_specify=off  T_I_nominal_unit=K  T_I_nominal_value=1  RH_I_specify=off  RH_I_priority=High  RH_I=0  RH_I_nominal_specify=off  RH_I_nominal_unit=1  RH_I_nominal_value=1  x_w_I_specify=off  x_w_I_priority=None  x_w_I=0  x_w_I_nominal_specify=off  x_w_I_nominal_unit=1  x_w_I_nominal_value=1  y_w_I_specify=off  y_w_I_priority=None  y_w_I=0  y_w_I_nominal_specify=off  y_w_I_nominal_unit=1  y_w_I_nominal_value=1  HR_I_specify=off  HR_I_priority=None  HR_I=0  HR_I_nominal_specify=off  HR_I_nominal_unit=1  HR_I_nominal_value=1  x_g_I_specify=off  x_g_I_priority=High  x_g_I=300  x_g_I_nominal_specify=off  x_g_I_nominal_unit=1  x_g_I_nominal_value=1  y_g_I_specify=on  y_g_I_priority=None  y_g_I=300  y_g_I_nominal_specify=off  y_g_I_nominal_unit=1  y_g_I_nominal_value=1
      settings: SourceProductBaseCode=SS  InternalSimscapePortConfiguration="{\"Bottom\":[],\"Left\":[{\"id\":\"A\",\"label\":\"A\",\"type\":\"foundation.moist_air.moist_air\"},{\"id\":\"B\",\"label\":\"B\",\"type\":\"foundation.moist_air.moist_air\"},{\"id\":\"C\",\"label\":\"C\",\"type\":\"foundation.moist_air.moist_air\"}],\"Right\":[{\"id\":\"W\",\"label\":\"W\",\"type\":\"output\"},{\"id\":\"F\",\"label\":\"F\",\"type\":\"output\"},{\"id\":\"H\",\"label\":\"H\",\"type\":\"foundation.thermal.thermal\"},{\"id\":\"S\",\"label\":\"S\",\"type\":\"foundation.moist_air.moist_air_source\"}],\"Top\":[]}"
  Constant2 : Constant
  Controlled Reservoir (MA)1 : fl_lib/Moist Air/Elements/Controlled Reservoir (MA)  moisture_spec=foundation.enum.moisture_spec.relative_humidity  trace_gas_spec=foundation.enum.trace_gas_spec.mole_fraction  RH_ws=1  area_A=duct_area m^2  input_error_spec=foundation.enum.input_range_error.warn
      settings: SourceProductBaseCode=SS  InternalSimscapePortConfiguration="{\"Bottom\":[],\"Left\":[{\"id\":\"A\",\"label\":\"A\",\"type\":\"foundation.moist_air.moist_air\"}],\"Right\":[{\"id\":\"T\",\"label\":\"T\",\"type\":\"input\"},{\"id\":\"P\",\"label\":\"P\",\"type\":\"input\"},{\"id\":\"W\",\"label\":\"W\",\"type\":\"input\"},{\"id\":\"G\",\"label\":\"G\",\"type\":\"input\"}],\"Top\":[]}"
  Controlled Reservoir (MA)2 : fl_lib/Moist Air/Elements/Controlled Reservoir (MA)  moisture_spec=foundation.enum.moisture_spec.relative_humidity  trace_gas_spec=foundation.enum.trace_gas_spec.mole_fraction  RH_ws=1  area_A=duct_area m^2  input_error_spec=foundation.enum.input_range_error.warn
      settings: SourceProductBaseCode=SS  InternalSimscapePortConfiguration="{\"Bottom\":[],\"Left\":[{\"id\":\"A\",\"label\":\"A\",\"type\":\"foundation.moist_air.moist_air\"}],\"Right\":[{\"id\":\"T\",\"label\":\"T\",\"type\":\"input\"},{\"id\":\"P\",\"label\":\"P\",\"type\":\"input\"},{\"id\":\"W\",\"label\":\"W\",\"type\":\"input\"},{\"id\":\"G\",\"label\":\"G\",\"type\":\"input\"}],\"Top\":[]}"
  Door Area : Gain  Gain=door_area
  Gain : Gain  Gain=1e6
  Local Restriction (MA) : fl_lib/Moist Air/Elements/Local Restriction (MA)  restriction_type=foundation.enum.restriction_type.variable  restriction_area=0.5 * duct_area m^2  min_area=1e-10 m^2  max_area=0.5*duct_area m^2  area=duct_area m^2  Cd=0.8  B_lam=0.999
      settings: SourceProductBaseCode=SS
  Local Restriction (MA)1 : fl_lib/Moist Air/Elements/Local Restriction (MA)  restriction_type=foundation.enum.restriction_type.fixed  restriction_area=0.5 * duct_area m^2  min_area=1e-10 m^2  max_area=0.5*duct_area m^2  area=duct_area m^2  Cd=0.8  B_lam=0.999
      settings: SourceProductBaseCode=SS  InternalSimscapePortConfiguration="{\"Bottom\":[],\"Left\":[{\"id\":\"A\",\"label\":\"A\",\"type\":\"foundation.moist_air.moist_air\"}],\"Right\":[{\"id\":\"B\",\"label\":\"B\",\"type\":\"foundation.moist_air.moist_air\"}],\"Top\":[]}"
  Measurement Selector (MA) : fl_lib/Moist Air/Sensors/Measurement Selector (MA)  moisture_spec=foundation.enum.moisture_spec.relative_humidity  trace_gas_spec=foundation.enum.trace_gas_spec.mole_fraction
      settings: SourceProductBaseCode=SS
  Occupant CO2 Gain : fl_lib/Moist Air/Sources/Moisture & Trace Gas Sources/Trace Gas Source (MA)  trace_gas_mass_flow=CO2_occupant * N_occupant g/s  temperature_spec=2  trace_gas_temperature=T_occupant degC
      settings: SourceProductBaseCode=SS  InternalSimscapePortConfiguration="{\"Bottom\":[],\"Left\":[{\"id\":\"S\",\"label\":\"S\",\"type\":\"foundation.moist_air.moist_air_source\"}],\"Right\":[],\"Top\":[]}"
  Occupant Moisture Gain : fl_lib/Moist Air/Sources/Moisture & Trace Gas Sources/Moisture Source (MA)  moisture_source_spec=foundation.enum.moisture_source_spec.vapor  moisture_mass_flow=W_occupant * N_occupant g/s  temperature_spec=2  moisture_temperature=T_occupant degC
      settings: SourceProductBaseCode=SS  InternalSimscapePortConfiguration="{\"Bottom\":[],\"Left\":[{\"id\":\"S\",\"label\":\"S\",\"type\":\"foundation.moist_air.moist_air_source\"}],\"Right\":[],\"Top\":[]}"
  PS-Simulink Converter : nesl_utility/PS-Simulink Converter  PhysicalDomain=network_engine_domain  SubClassName=ps_output  LeftPortType=input  RightPortType=output  PseudoPeriodic=off  Frequencies=[]  Unit=1  AffineConversion=on
  PS-Simulink Converter1 : nesl_utility/PS-Simulink Converter  PhysicalDomain=network_engine_domain  SubClassName=ps_output  LeftPortType=input  RightPortType=output  PseudoPeriodic=off  Frequencies=[]  Unit=degC  AffineConversion=on
  PS-Simulink Converter2 : nesl_utility/PS-Simulink Converter  PhysicalDomain=network_engine_domain  SubClassName=ps_output  LeftPortType=input  RightPortType=output  PseudoPeriodic=off  Frequencies=[]  Unit=1  AffineConversion=on
  Scope : Scope
  Simulink-PS Converter : nesl_utility/Simulink-PS Converter  PhysicalDomain=network_engine_domain  SubClassName=ps_input  LeftPortType=input  RightPortType=output  PseudoPeriodic=off  Frequencies=[]  NoiseDistribution=none  NoiseParameters=[]  Unit=1  AffineConversion=off  FilteringAndDerivatives=provide  SimscapeFilterOrder=1  InputFilterTimeConstant=0.001  UdotUserProvided=0
  Simulink-PS Converter1 : nesl_utility/Simulink-PS Converter  PhysicalDomain=network_engine_domain  SubClassName=ps_input  LeftPortType=input  RightPortType=output  PseudoPeriodic=off  Frequencies=[]  NoiseDistribution=none  NoiseParameters=[]  Unit=1  AffineConversion=off  FilteringAndDerivatives=provide  SimscapeFilterOrder=1  InputFilterTimeConstant=0.001  UdotUserProvided=0
  Simulink-PS Converter4 : nesl_utility/Simulink-PS Converter  PhysicalDomain=network_engine_domain  SubClassName=ps_input  LeftPortType=input  RightPortType=output  PseudoPeriodic=off  Frequencies=[]  NoiseDistribution=none  NoiseParameters=[]  Unit=degC  AffineConversion=on  FilteringAndDerivatives=provide  SimscapeFilterOrder=1  InputFilterTimeConstant=0.001  UdotUserProvided=0
  Simulink-PS Converter5 : nesl_utility/Simulink-PS Converter  PhysicalDomain=network_engine_domain  SubClassName=ps_input  LeftPortType=input  RightPortType=output  PseudoPeriodic=off  Frequencies=[]  NoiseDistribution=none  NoiseParameters=[]  Unit=atm  AffineConversion=on  FilteringAndDerivatives=provide  SimscapeFilterOrder=1  InputFilterTimeConstant=0.001  UdotUserProvided=0
  Simulink-PS Converter6 : nesl_utility/Simulink-PS Converter  PhysicalDomain=network_engine_domain  SubClassName=ps_input  LeftPortType=input  RightPortType=output  PseudoPeriodic=off  Frequencies=[]  NoiseDistribution=none  NoiseParameters=[]  Unit=m^2  AffineConversion=off  FilteringAndDerivatives=provide  SimscapeFilterOrder=1  InputFilterTimeConstant=0.001  UdotUserProvided=0
  Thermal Resistance 4 : Subsystem  mask(Zone Thermal Resistance){zone_length=building_length / 2, zone_width=building_width / 2, zone_height=building_height / 2, wall_thickness=wall_thickness, wall_density=wall_density, wall_specific_heat=wall_specific_heat, wall_conductivity=wall_conductivity, wall_heat_transfer_coeff_internal=wall_heat_transfer_coeff_internal, wall_heat_transfer_coeff_external=wall_heat_transfer_coeff_external, wall_initial_temperature=initial_temperature, roof_thickness=roof_thickness, roof_density=roof_density, roof_specific_heat=roof_specific_heat, roof_conductivity=roof_conductivity, roof_heat_transfer_coeff_internal=roof_heat_transfer_coeff_internal, roof_heat_transfer_coeff_external=roof_heat_transfer_coeff_external, roof_initial_temperature=initial_temperature, floor_thickness=floor_thickness, floor_conductivity=floor_conductivity, floor_heat_transfer_coeff_internal=floor_heat_transfer_coeff_internal, ground_temperature=ground_temperature}
      mask prompts: zone_length "Zone length (m)"; zone_width "Zone width (m)"; zone_height "Zone height (m)"; wall_thickness "Thickness (m)"; wall_density "Density (kg/m^3)"; wall_specific_heat "Specific heat (J/(kg*K))"; wall_conductivity "Thermal conductivity (W/(m*K))"; wall_heat_transfer_coeff_internal "Internal heat transfer coefficient (W/(m^2*K))"; wall_heat_transfer_coeff_external "External heat transfer coefficient (W/(m^2*K))"; wall_initial_temperature "Initial temperature (degC)"; roof_thickness "Thickness (m)"; roof_density "Density (kg/m^3)"; roof_specific_heat "Specific heat (J/(kg*K))"; roof_conductivity "Thermal conductivity (W/(m*K))"; roof_heat_transfer_coeff_internal "Internal heat transfer coefficient (W/(m^2*K))"; roof_heat_transfer_coeff_external "External heat transfer coefficient (W/(m^2*K))"; roof_initial_temperature "Initial temperature (degC)"; floor_thickness "Thickness (m)"; floor_conductivity "Thermal conductivity (W/(m*K))"; floor_heat_transfer_coeff_internal "Internal heat transfer coefficient (W/(m^2*K))"; ground_temperature "Ground temperature (degC)"
      mask help: This subsystem models the thermal resistances of the wall and of the roof between the zone and the external environment. It also models the thermal resistance of the floor between the zone and the ground.
      mask init:
      | wall_area = zone_height * (zone_length + zone_width);
      | roof_area = zone_length * zone_width;
      | floor_area = zone_length * zone_width;
      mask DialogControl TabGeometry Prompt: Geometry
      mask DialogControl TabWall Prompt: Wall
      mask DialogControl TabRoof Prompt: Roof
      mask DialogControl TabFloor Prompt: Floor
  co2_env : Constant  Value=y_co2_env
  IN : PMIOPort  Side=Right
  OUT : PMIOPort  Port=2  Side=Left
  tag scope: RH_room=global, T2=global, co2_room=global
  wires:
  Constant2/1 -> Simulink-PS Converter5/1
  [door] -> Door Area/1
  [T_ext] -> Simulink-PS Converter4/1
  [T_ext] -> Thermal Resistance 4/1(Ext)
  Door Area/1 -> Simulink-PS Converter6/1
  co2_env/1 -> Simulink-PS Converter/1
  Gain/1 -> [co2_room]
  PS-Simulink Converter/1 -> Gain/1
  PS-Simulink Converter1/1 -> [T2]
  Constant/1 -> Simulink-PS Converter1/1
  PS-Simulink Converter2/1 -> [RH_room], Scope/1
  connections:
  Simulink-PS Converter5/RConn1 -- Controlled Reservoir (MA)2/RConn2 -- Controlled Reservoir (MA)1/RConn2
  Local Restriction (MA)/LConn2 -- Simulink-PS Converter6/RConn1
  Controlled Reservoir (MA)1/LConn1 -- Local Restriction (MA)/LConn1
  Thermal Resistance 4/RConn1 -- Constant Volume Chamber (MA)1/RConn3
  Local Restriction (MA)/RConn1 -- Constant Volume Chamber (MA)1/LConn1
  Simulink-PS Converter4/RConn1 -- Controlled Reservoir (MA)1/RConn1 -- Controlled Reservoir (MA)2/RConn1
  Constant Volume Chamber (MA)1/LConn2 -- OUT/RConn1 -- Local Restriction (MA)1/LConn1
  IN/RConn1 -- Constant Volume Chamber (MA)1/LConn3
  Occupant Moisture Gain/LConn1 -- Occupant CO2 Gain/LConn1 -- Constant Volume Chamber (MA)1/RConn4
  Local Restriction (MA)1/RConn1 -- Controlled Reservoir (MA)2/LConn1
  Simulink-PS Converter/RConn1 -- Controlled Reservoir (MA)1/RConn4 -- Controlled Reservoir (MA)2/RConn4
  Constant Volume Chamber (MA)1/RConn2 -- Measurement Selector (MA)/LConn1
  Measurement Selector (MA)/RConn4 -- PS-Simulink Converter/LConn1
  Measurement Selector (MA)/RConn2 -- PS-Simulink Converter1/LConn1
  Simulink-PS Converter1/RConn1 -- Controlled Reservoir (MA)1/RConn3 -- Controlled Reservoir (MA)2/RConn3
  Measurement Selector (MA)/RConn3 -- PS-Simulink Converter2/LConn1

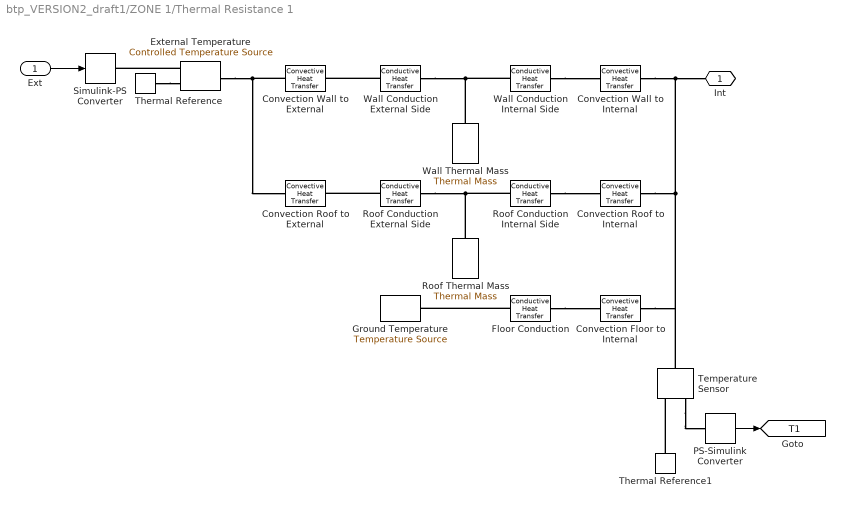
== system btp_VERSION2_draft1/ZONE 1/Thermal Resistance 1 ==
  Ext : Inport
  Convection Floor to Internal : fl_lib/Thermal/Thermal Elements/Convective Heat Transfer  area=floor_area m^2  heat_tr_coeff=floor_heat_transfer_coeff_internal W/(m^2 * K)  T_specify=off  T_priority=None  T=0 K  T_nominal_specify=off  T_nominal_unit=K  T_nominal_value=1  Q_specify=off  Q_priority=None  Q=0 W  Q_nominal_specify=off  Q_nominal_unit=W  Q_nominal_value=1
  Convection Roof to External : fl_lib/Thermal/Thermal Elements/Convective Heat Transfer  area=roof_area m^2  heat_tr_coeff=roof_heat_transfer_coeff_external W/(m^2 * K)  T_specify=off  T_priority=None  T=0 K  T_nominal_specify=off  T_nominal_unit=K  T_nominal_value=1  Q_specify=off  Q_priority=None  Q=0 W  Q_nominal_specify=off  Q_nominal_unit=W  Q_nominal_value=1
  Convection Roof to Internal : fl_lib/Thermal/Thermal Elements/Convective Heat Transfer  area=roof_area m^2  heat_tr_coeff=roof_heat_transfer_coeff_internal W/(m^2 * K)  T_specify=off  T_priority=None  T=0 K  T_nominal_specify=off  T_nominal_unit=K  T_nominal_value=1  Q_specify=off  Q_priority=None  Q=0 W  Q_nominal_specify=off  Q_nominal_unit=W  Q_nominal_value=1
  Convection Wall to External : fl_lib/Thermal/Thermal Elements/Convective Heat Transfer  area=wall_area m^2  heat_tr_coeff=wall_heat_transfer_coeff_external W/(m^2 * K)  T_specify=off  T_priority=None  T=0 K  T_nominal_specify=off  T_nominal_unit=K  T_nominal_value=1  Q_specify=off  Q_priority=None  Q=0 W  Q_nominal_specify=off  Q_nominal_unit=W  Q_nominal_value=1
  Convection Wall to Internal : fl_lib/Thermal/Thermal Elements/Convective Heat Transfer  area=wall_area m^2  heat_tr_coeff=wall_heat_transfer_coeff_internal W/(m^2 * K)  T_specify=off  T_priority=None  T=0 K  T_nominal_specify=off  T_nominal_unit=K  T_nominal_value=1  Q_specify=off  Q_priority=None  Q=0 W  Q_nominal_specify=off  Q_nominal_unit=W  Q_nominal_value=1
  External Temperature : fl_lib/Thermal/Thermal Sources/Controlled Temperature Source
  Floor Conduction : fl_lib/Thermal/Thermal Elements/Conductive Heat Transfer  area=floor_area m^2  thickness=floor_thickness m  th_cond=floor_conductivity W/(m*K)  T_specify=off  T_priority=None  T=0 K  T_nominal_specify=off  T_nominal_unit=K  T_nominal_value=1  Q_specify=off  Q_priority=None  Q=0 W  Q_nominal_specify=off  Q_nominal_unit=W  Q_nominal_value=1
  Ground Temperature : fl_lib/Thermal/Thermal Sources/Temperature Source  temperature=ground_temperature degC
  PS-Simulink Converter : nesl_utility/PS-Simulink Converter  PhysicalDomain=network_engine_domain  SubClassName=ps_output  LeftPortType=input  RightPortType=output  PseudoPeriodic=off  Frequencies=[]  Unit=degC  AffineConversion=on
  Roof Conduction External Side : fl_lib/Thermal/Thermal Elements/Conductive Heat Transfer  area=roof_area m^2  thickness=roof_thickness / 2 m  th_cond=roof_conductivity W/(m*K)  T_specify=off  T_priority=None  T=0 K  T_nominal_specify=off  T_nominal_unit=K  T_nominal_value=1  Q_specify=off  Q_priority=None  Q=0 W  Q_nominal_specify=off  Q_nominal_unit=W  Q_nominal_value=1
  Roof Conduction Internal Side : fl_lib/Thermal/Thermal Elements/Conductive Heat Transfer  area=roof_area m^2  thickness=roof_thickness / 2 m  th_cond=roof_conductivity W/(m*K)  T_specify=off  T_priority=None  T=0 K  T_nominal_specify=off  T_nominal_unit=K  T_nominal_value=1  Q_specify=off  Q_priority=None  Q=0 W  Q_nominal_specify=off  Q_nominal_unit=W  Q_nominal_value=1
  Roof Thermal Mass : fl_lib/Thermal/Thermal Elements/Thermal Mass  mass=roof_area * roof_thickness * wall_density kg  sp_heat=roof_specific_heat J/kg/K  T_specify=on  T_priority=High  T=roof_initial_temperature degC  T_nominal_specify=off  T_nominal_unit=K  T_nominal_value=1  Q_specify=off  Q_priority=None  Q=0 W  Q_nominal_specify=off  Q_nominal_unit=W  Q_nominal_value=1
  Simulink-PS Converter : nesl_utility/Simulink-PS Converter  PhysicalDomain=network_engine_domain  SubClassName=ps_input  LeftPortType=input  RightPortType=output  PseudoPeriodic=off  Frequencies=[]  NoiseDistribution=none  NoiseParameters=[]  Unit=degC  AffineConversion=on  FilteringAndDerivatives=provide  SimscapeFilterOrder=1  InputFilterTimeConstant=0.001  UdotUserProvided=0
  Temperature Sensor : fl_lib/Thermal/Thermal Sensors/Temperature Sensor
  Thermal Reference : fl_lib/Thermal/Thermal Elements/Thermal Reference
  Thermal Reference1 : fl_lib/Thermal/Thermal Elements/Thermal Reference
  Wall Conduction External Side : fl_lib/Thermal/Thermal Elements/Conductive Heat Transfer  area=wall_area m^2  thickness=wall_thickness / 2 m  th_cond=wall_conductivity W/(m*K)  T_specify=off  T_priority=None  T=0 K  T_nominal_specify=off  T_nominal_unit=K  T_nominal_value=1  Q_specify=off  Q_priority=None  Q=0 W  Q_nominal_specify=off  Q_nominal_unit=W  Q_nominal_value=1
  Wall Conduction Internal Side : fl_lib/Thermal/Thermal Elements/Conductive Heat Transfer  area=wall_area m^2  thickness=wall_thickness / 2 m  th_cond=wall_conductivity W/(m*K)  T_specify=off  T_priority=None  T=0 K  T_nominal_specify=off  T_nominal_unit=K  T_nominal_value=1  Q_specify=off  Q_priority=None  Q=0 W  Q_nominal_specify=off  Q_nominal_unit=W  Q_nominal_value=1
  Wall Thermal Mass : fl_lib/Thermal/Thermal Elements/Thermal Mass  mass=wall_area * wall_thickness * wall_density kg  sp_heat=wall_specific_heat J/kg/K  T_specify=on  T_priority=High  T=wall_initial_temperature degC  T_nominal_specify=off  T_nominal_unit=K  T_nominal_value=1  Q_specify=off  Q_priority=None  Q=0 W  Q_nominal_specify=off  Q_nominal_unit=W  Q_nominal_value=1
  Int : PMIOPort  Side=Right
  tag scope: T1=global
  wires:
  Ext/1 -> Simulink-PS Converter/1
  PS-Simulink Converter/1 -> [T1]
  connections:
  External Temperature/RConn1 -- Simulink-PS Converter/RConn1
  Wall Conduction Internal Side/RConn1 -- Convection Wall to Internal/LConn1
  Convection Roof to Internal/RConn1 -- Convection Floor to Internal/RConn1 -- Temperature Sensor/LConn1 -- Convection Wall to Internal/RConn1 -- Int/RConn1
  External Temperature/LConn1 -- Convection Wall to External/LConn1 -- Convection Roof to External/LConn1
  Wall Conduction External Side/LConn1 -- Convection Wall to External/RConn1
  Wall Thermal Mass/LConn1 -- Wall Conduction Internal Side/LConn1 -- Wall Conduction External Side/RConn1
  Roof Thermal Mass/LConn1 -- Roof Conduction Internal Side/LConn1 -- Roof Conduction External Side/RConn1
  Roof Conduction External Side/LConn1 -- Convection Roof to External/RConn1
  Roof Conduction Internal Side/RConn1 -- Convection Roof to Internal/LConn1
  Floor Conduction/RConn1 -- Convection Floor to Internal/LConn1
  Floor Conduction/LConn1 -- Ground Temperature/LConn1
  Thermal Reference1/LConn1 -- Temperature Sensor/RConn1
  Temperature Sensor/RConn2 -- PS-Simulink Converter/LConn1
  Thermal Reference/LConn1 -- External Temperature/RConn2
